simulink model "dc_motor_from_A_to_B"  (R2015a)
settings: Solver=ode45  StartTime=0.0  StopTime=1  MaxStep=1/10000  RelTol=1e-3
values from neighbouring files (symbols this model uses):
  j = 0.575/1000    (= 0.000575)    [motor_a2b_param.m]    (also in motor_param.m = 0.02)
  k = 0.93    [motor_a2b_param.m]    (also in motor_param.m = 0.796; para.m = 0.5)
  la = 25/1000    (= 0.025)    [motor_a2b_param.m]    (also in motor_param.m = 0.01)
  ra = 7.8    [motor_a2b_param.m]    (also in motor_param.m = 0.78)
libraries: powerlib x10
settings Model: Creator=Windows 10  LastModifiedBy=Windows 10

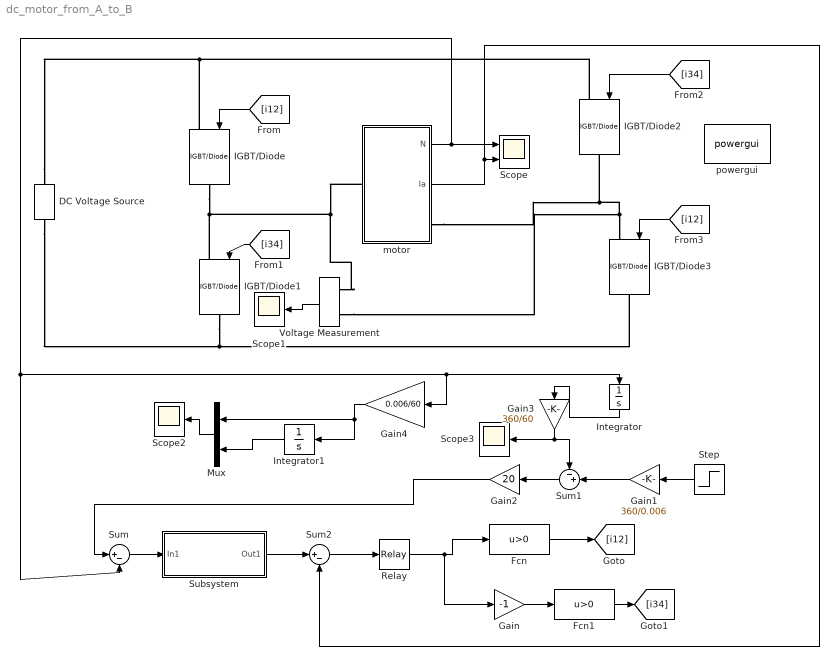
== system dc_motor_from_A_to_B ==
  DC Voltage Source : powerlib/Electrical Sources/DC Voltage Source  Amplitude=310  Measurements=None
  Fcn : Fcn  Expr=u>0
  Fcn1 : Fcn  Expr=u>0
  Gain : Gain  Gain=-1
  Gain1 : Gain  Gain=360/0.006
  Gain2 : Gain  Gain=20
  Gain3 : Gain  Gain=360/60
  Gain4 : Gain  Gain=0.006/60
  IGBT/Diode{,1..3} (4 alike) : powerlib/Power Electronics/IGBT//Diode  Ron=1e-3  Rs=1e5  Cs=inf  Measurements=off
  Integrator : Integrator
  Integrator1 : Integrator
  Mux : Mux  Inputs=2
  Relay : Relay  OnSwitchValue=1  OffSwitchValue=-1  OffOutputValue=-1
  Scope : Scope  NumInputPorts=2
      settings: YMin=-5~-5  YMax=5~5
  Scope1 : Scope
  Scope2 : Scope
      settings: SaveName=ScopeData2
  Scope3 : Scope
      settings: SaveName=ScopeData3
  Step : Step  Time=0.5  Before=0.1  After=0  SampleTime=0
  Subsystem : Subsystem
  Sum : Sum  Inputs=|+-
  Sum1 : Sum  Inputs=-+|
  Sum2 : Sum  Inputs=|+-
  Voltage Measurement : powerlib/Measurements/Voltage Measurement  PhasorSimulation=off  OutputType=Complex  PSBequivalent=0
  "motor " : Subsystem
  powergui : powerlib/powergui  Priority=1  SimulationMode=Continuous  SolverType=Tustin/Backward Euler (TBE)  SampleTime=50e-6  frequency=60  SPID=off  DisableSnubberDevices=off  DisableRonSwitches=off  DisableVfSwitches=off  SwTol=0  DisplayEquations=off  Interpol=off  methode=off  Ts=100  FunctionMessages=off  echomessages=off  HookPort=off  EnableUseOfTLC=off  x0status=blocks  frequencyindice=0  Pbase=100e6  ErrMax=1e-4  Iterations=50  UnitsV=kV  UnitsW=MW  buscounter=0  RestoreLinks=warning  ResistiveCurrentMeasurement=off  Frange=[0:2:500]  Ylog=off  Xlog=on  ShowGrid=off  save=off  variable=ZData  structure=0  ZoomFFT=off  StartTime=0.0  cycles=1  DisplayStyle=1  fundamental=60  FreqAxis=off  MaxFrequency=1000  frequencyindicesteady=1  RmsSteady=1  display=off
  wires:
  Voltage Measurement/1 -> Scope1/1
  Sum/1 -> Subsystem/1(In1)
  "motor "/1(N) -> Sum/2, Integrator/1, Gain4/1, Scope/1
  "motor "/2("Ia ") -> Sum2/2, Scope/2
  Gain/1 -> Fcn1/1
  Fcn1/1 -> [i34]
  Fcn/1 -> [i12]
  [i12] -> IGBT/Diode/1
  [i34] -> IGBT/Diode1/1
  [i34] -> IGBT/Diode2/1
  [i12] -> IGBT/Diode3/1
  Subsystem/1(Out1) -> Sum2/1
  Sum2/1 -> Relay/1
  Relay/1 -> Gain/1, Fcn/1
  Gain1/1 -> Sum1/2
  Step/1 -> Gain1/1
  Sum1/1 -> Gain2/1
  Integrator/1 -> Gain3/1
  Gain4/1 -> Mux/1, Integrator1/1
  Integrator1/1 -> Mux/2
  Mux/1 -> Scope2/1
  Gain2/1 -> Sum/1
  Gain3/1 -> Sum1/1, Scope3/1
  connections:
  "motor "/LConn1 -- Voltage Measurement/LConn1 -- IGBT/Diode1/LConn1 -- IGBT/Diode/RConn1
  DC Voltage Source/RConn1 -- IGBT/Diode2/LConn1 -- IGBT/Diode/LConn1
  Voltage Measurement/LConn2 -- "motor "/RConn1 -- IGBT/Diode2/RConn1 -- IGBT/Diode3/LConn1
  DC Voltage Source/LConn1 -- IGBT/Diode3/RConn1 -- IGBT/Diode1/RConn1

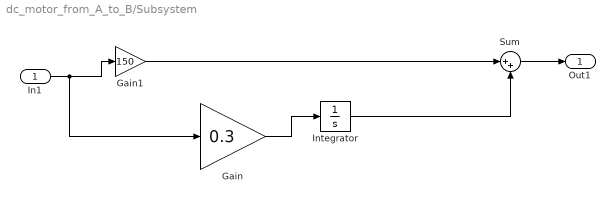
== system dc_motor_from_A_to_B/Subsystem ==
  In1 : Inport
  Gain : Gain  Gain=0.3
  Gain1 : Gain  Gain=150
  Integrator : Integrator
  Sum : Sum  Inputs=|++
  Out1 : Outport
  wires:
  In1/1 -> Gain/1, Gain1/1
  Gain/1 -> Integrator/1
  Integrator/1 -> Sum/2
  Gain1/1 -> Sum/1
  Sum/1 -> Out1/1

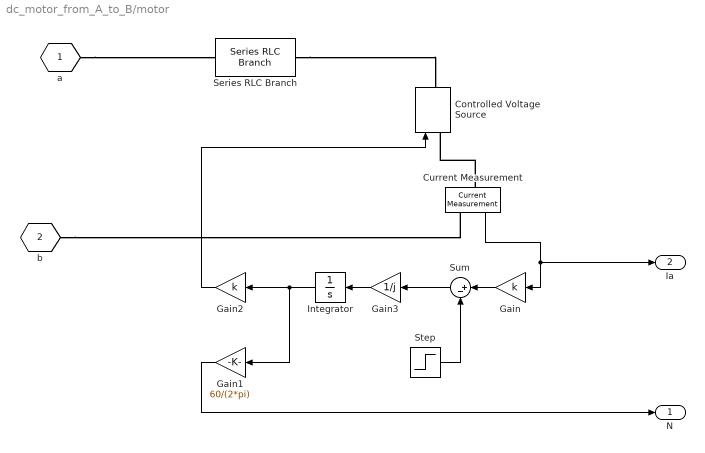
== system dc_motor_from_A_to_B/motor  ==
  Controlled Voltage Source : powerlib/Electrical Sources/Controlled Voltage Source  Initialize=on  Source_Type=AC  Amplitude=0  Phase=0  Frequency=0  Measurements=None
  Current Measurement : powerlib/Measurements/Current Measurement  PhasorSimulation=off  OutputType=Complex  PSBequivalent=0
  Gain : Gain  Gain=k
  Gain1 : Gain  Gain=60/(2*pi)
  Gain2 : Gain  Gain=k
  Gain3 : Gain  Gain=1/j
  Integrator : Integrator
  Series RLC Branch : powerlib/Elements/Series RLC Branch  LConnTagsString=__new0  RConnTagsString=__new0  BranchType=RL  Resistance=ra  Inductance=la  SetiL0=on  InitialCurrent=0  Capacitance=1e-6  Setx0=off  InitialVoltage=0  Measurements=None
  Step : Step  Time=0.5  Before=2  After=-2  SampleTime=0
  Sum : Sum  Inputs=|+-
  a : PMIOPort  Tag=PMCPort  Port=1  Side=Left
  "b " : PMIOPort  Tag=PMCPort  Port=2  Side=Right
  N : Outport
  "Ia " : Outport  Port=2
  wires:
  Current Measurement/1 -> "Ia "/1, Gain/1
  Gain/1 -> Sum/1
  Step/1 -> Sum/2
  Sum/1 -> Gain3/1
  Gain3/1 -> Integrator/1
  Integrator/1 -> Gain1/1, Gain2/1
  Gain2/1 -> Controlled Voltage Source/1
  Gain1/1 -> N/1
  connections:
  a/RConn1 -- Series RLC Branch/LConn1
  Series RLC Branch/RConn1 -- Controlled Voltage Source/RConn1
  Current Measurement/LConn1 -- Controlled Voltage Source/LConn1
  "b "/RConn1 -- Current Measurement/RConn1
